simulink model "MySimModel"  (R2024b)
settings: Solver=VariableStepAuto  StartTime=0.0  StopTime=10.0  RelTol=1e-3
settings Model: Creator=xinxing  LastModifiedBy=xinxing

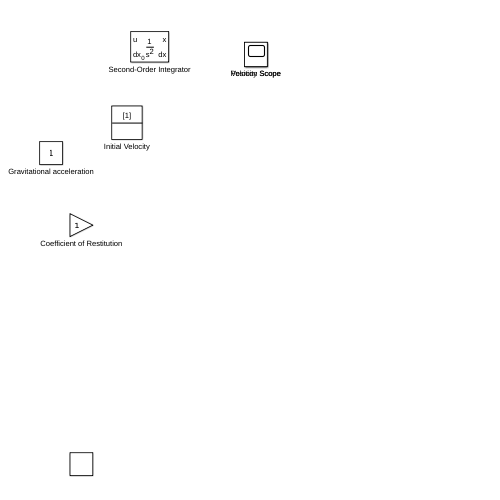
[thumbnail: Simulink's stored preview of the top-level diagram]
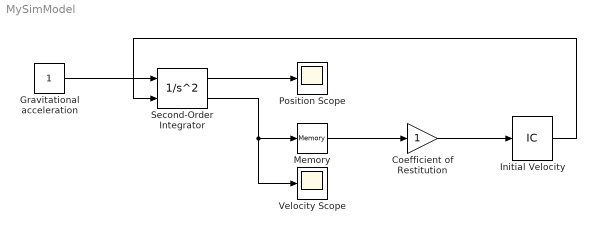
== system MySimModel ==
  Coefficient of Restitution : Gain
  Gravitational acceleration : Constant
  Initial Velocity : InitialCondition
  Memory : Memory
  Position Scope : Scope
  Second-Order Integrator : SecondOrderIntegrator  ICSourceDXDT=external
  Velocity Scope : Scope
  wires:
  Initial Velocity/1 -> Second-Order Integrator/2
  Coefficient of Restitution/1 -> Initial Velocity/1
  Memory/1 -> Coefficient of Restitution/1
  Second-Order Integrator/2 -> Memory/1, Velocity Scope/1
  Second-Order Integrator/1 -> Position Scope/1
  Gravitational acceleration/1 -> Second-Order Integrator/1
